simulink model "exhaust_system"  (R2015b)
settings: Solver=VariableStepAuto  StartTime=0.0  StopTime=10.0  RelTol=1e-3
values from neighbouring files (symbols this model uses):
  k = 1    [testfile.m]
  m_dot_exh_test = m_dot_fc_test+m_dot_ac_test    [testfile.m]
  p_em_test = p_em(k)    [testfile.m]
  T_em_test = T_em(k)    [testfile.m]
undefined symbols (not defined in the file or in its folder): C_2, p_amb, R_exh, T_0, V_em
settings Model: Creator=nicgr354  LastModifiedBy=nicgr354

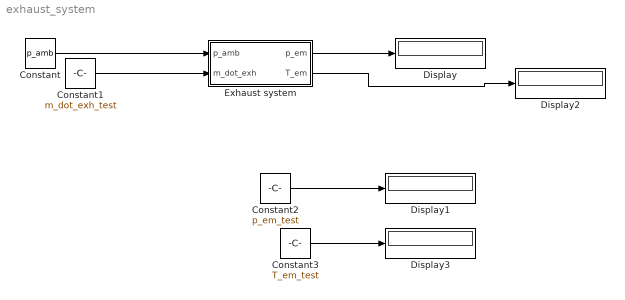
== system exhaust_system ==
  Constant : Constant  Value=p_amb
  Constant1 : Constant  Value=m_dot_exh_test
  Constant2 : Constant  Value=p_em_test
  Constant3 : Constant  Value=T_em_test
  Display{,1..3} (4 alike) : Display
  Exhaust system : Subsystem
  wires:
  Exhaust system/1(p_em) -> Display/1
  Exhaust system/2(T_em) -> Display2/1
  Constant/1 -> Exhaust system/1(p_amb)
  Constant1/1 -> Exhaust system/2(m_dot_exh)
  Constant2/1 -> Display1/1
  Constant3/1 -> Display3/1

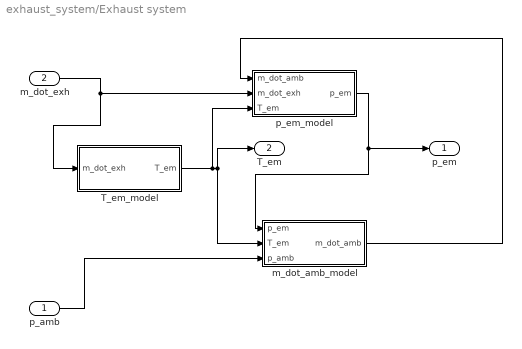
== system exhaust_system/Exhaust system ==
  p_amb : Inport
  m_dot_exh : Inport  Port=2
  T_em_model : Subsystem
  "m_dot_amb_model " : Subsystem
  p_em_model : Subsystem
  p_em : Outport
  T_em : Outport  Port=2
  wires:
  p_amb/1 -> "m_dot_amb_model "/3(p_amb)
  p_em_model/1(p_em) -> "m_dot_amb_model "/1(p_em), p_em/1
  T_em_model/1(T_em) -> p_em_model/3(T_em), "m_dot_amb_model "/2(T_em), T_em/1
  m_dot_exh/1 -> p_em_model/2(m_dot_exh), T_em_model/1(m_dot_exh)
  "m_dot_amb_model "/1(m_dot_amb) -> p_em_model/1(m_dot_amb)

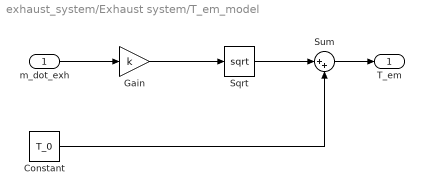
== system exhaust_system/Exhaust system/T_em_model ==
  m_dot_exh : Inport
  Constant : Constant  Value=T_0
  Gain : Gain  Gain=k
  Sqrt : Sqrt  SaturateOnIntegerOverflow=on
  Sum : Sum  Inputs=|++
  T_em : Outport
  wires:
  Sqrt/1 -> Sum/1
  m_dot_exh/1 -> Gain/1
  Gain/1 -> Sqrt/1
  Constant/1 -> Sum/2
  Sum/1 -> T_em/1

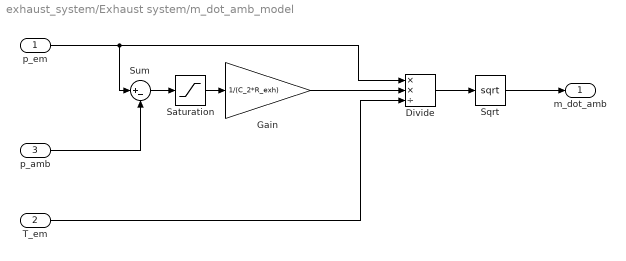
== system exhaust_system/Exhaust system/m_dot_amb_model  ==
  p_em : Inport
  T_em : Inport  Port=2
  p_amb : Inport  Port=3
  Divide : Product  Inputs=**/
  Gain : Gain  Gain=1/(C_2*R_exh)
  Saturation : Saturate  UpperLimit=inf  LowerLimit=0
  Sqrt : Sqrt  SaturateOnIntegerOverflow=on
  Sum : Sum  Inputs=|+-
  m_dot_amb : Outport
  wires:
  p_amb/1 -> Sum/2
  Sum/1 -> Saturation/1
  T_em/1 -> Divide/3
  p_em/1 -> Divide/1, Sum/1
  Gain/1 -> Divide/2
  Divide/1 -> Sqrt/1
  Sqrt/1 -> m_dot_amb/1
  Saturation/1 -> Gain/1

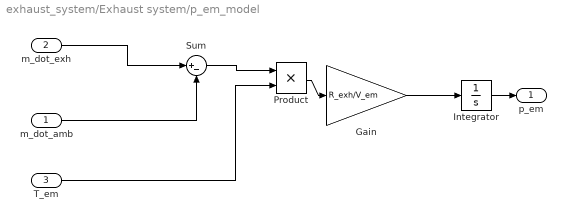
== system exhaust_system/Exhaust system/p_em_model ==
  m_dot_amb : Inport
  m_dot_exh : Inport  Port=2
  T_em : Inport  Port=3
  Gain : Gain  Gain=R_exh/V_em
  Integrator : Integrator  InitialCondition=p_amb
  Product : Product
  Sum : Sum  Inputs=|+-
  p_em : Outport
  wires:
  m_dot_exh/1 -> Sum/1
  m_dot_amb/1 -> Sum/2
  Sum/1 -> Product/1
  T_em/1 -> Product/2
  Product/1 -> Gain/1
  Gain/1 -> Integrator/1
  Integrator/1 -> p_em/1
